simulink model "ButtonLogic"  (R2023b)
settings: Solver=FixedStepDiscrete  StartTime=0.0  StopTime=inf  FixedStep=0.005  RelTol=1e-3  EnableMultiTasking=on
model workspace (MAT data in the model file):
  inSetButton = 0
undefined symbols (not defined in the file or in its folder): eStateName
libraries: simulink x5
(part 1 of 3)
settings Model: DataDictionary=ButtonLogicData.sldd  Creator=pkpam  LastModifiedBy=pkpam
settings SolverCC: AlgebraicLoopSolver=TrustRegion  AutoInsertRateTranBlk=on
settings DataIOCC: LimitDataPoints=on
settings OptimizationCC: DefaultUnderspecifiedDataType=single  ReuseModelBlockBuffer=off  PassReuseOutputArgsAs=Individual arguments  ZeroExternalMemoryAtStartup=off  ZeroInternalMemoryAtStartup=off  OptimizationLevel=level1  EfficientTunableParamExpr=on
settings DebuggingCC: ParameterTunabilityLossMsg=error  UnconnectedInputMsg=warning  UnconnectedOutputMsg=warning  UnconnectedLineMsg=warning  AssertControl=DisableAll  AllowSymbolicDim=off  SFUnexpectedBacktrackingDiag=warning  SFNoUnconditionalDefaultTransitionDiag=warning  SFExecutionAtInitializationDiag=none  ArithmeticOperatorsInVariantConditions=warning
settings ModelReferenceCC: EnableRefExpFcnMdlSchedulingChecks=on  ModelReferenceNumInstancesAllowed=Single
settings SFSimCC: SimUseLocalCustomCode=off  MATLABDynamicMemAlloc=off  CustomCodeUndefinedFunction=UseInterfaceOnly
settings RTWCC: Description=Embedded Coder  SystemTargetFile=ert.tlc  TemplateMakefile=ert_default_tmf  GenerateReport=on  RTWUseLocalCustomCode=off  Toolchain=LCC-win64 v2.4.1 | gmake (64-bit Windows)  DataTypeReplacement=CDataTypesFixedWidth  GenerateWebview=on  CheckMdlBeforeBuild=Warning  DLArmComputeVersion=19.05
settings CodeAppCC: ForceParamTrailComments=on  IgnoreCustomStorageClasses=off  OperatorAnnotations=on  SimulinkDataObjDesc=on  SFDataObjDesc=on  MATLABFcnDesc=on  InsertBlockDesc=on  StateflowObjectComments=on
settings ERTTargetCC: UtilityFuncGeneration=Shared location  GenerateSampleERTMain=on  SupportNonFinite=off  GenerateSharedConstants=off  MultiInstanceErrorCode=Warning  ERTCustomFileTemplate=example_file_process.tlc  GlobalDataDefinition=InSourceFile  ERTFilePackagingFormat=CompactWithDataFile  IndentSize=4  MaxIdInt64=INT64_MAX  MinIdInt64=INT64_MIN  MaxIdUint64=UINT64_MAX  MaxIdInt32=INT32_MAX  MinIdInt32=INT32_MIN  MaxIdUint32=UINT32_MAX  MaxIdInt16=INT16_MAX  MinIdInt16=INT16_MIN  MaxIdUint16=UINT16_MAX  MaxIdInt8=INT8_MAX  MinIdInt8=INT8_MIN  MaxIdUint8=UINT8_MAX
settings ConfigComp: CovMetricSettings=dw  CovSaveCumulativeToWorkspaceVar=on  CovSaveSingleToWorkspaceVar=on  CovExternalEMLEnable=off  CovSFcnEnable=off

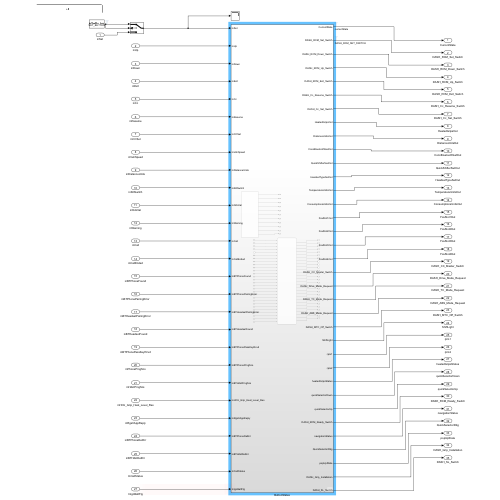
[thumbnail: Simulink's stored preview of the top-level diagram]
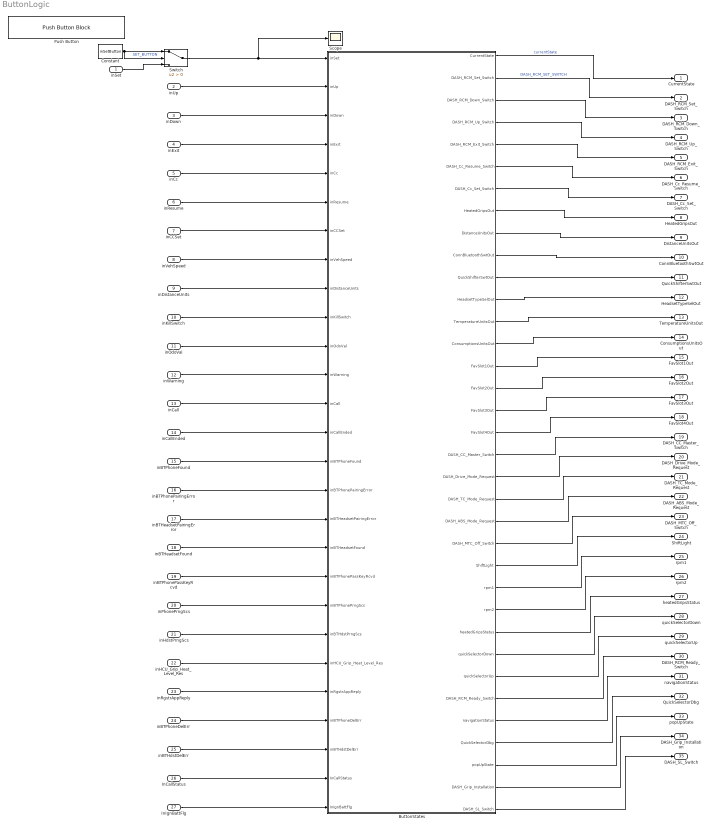
== system ButtonLogic ==
  inSet : Inport  OutDataTypeStr=boolean
  inUp : Inport  Port=2  OutDataTypeStr=boolean
  inDown : Inport  Port=3  OutDataTypeStr=boolean
  inExit : Inport  Port=4  OutDataTypeStr=boolean
  inCc : Inport  Port=5
  inResume : Inport  Port=6
  inCCSet : Inport  Port=7
  inVehSpeed : Inport  Port=8
  inDistanceUnits : Inport  Port=9  OutDataTypeStr=uint8
  inKillSwitch : Inport  Port=10  OutDataTypeStr=uint8
  inOdoVal : Inport  Port=11  OutDataTypeStr=uint32
  inWarning : Inport  Port=12
  inCall : Inport  Port=13
  inCallEnded : Inport  Port=14
  inBTPhoneFound : Inport  Port=15  OutDataTypeStr=boolean
  inBTPhonePairingError : Inport  Port=16  OutDataTypeStr=boolean
  inBTHeadsetPairingError : Inport  Port=17  OutDataTypeStr=boolean
  inBTHeadsetFound : Inport  Port=18  OutDataTypeStr=boolean
  inBTPhonePassKeyRcvd : Inport  Port=19  OutDataTypeStr=boolean
  inPhonePrngScs : Inport  Port=20  OutDataTypeStr=boolean
  inHdstPrngScs : Inport  Port=21  OutDataTypeStr=boolean
  inHCU_Grip_Heat_Level_Res : Inport  Port=22  OutDataTypeStr=boolean
  inRgstrAppReply : Inport  Port=23  OutDataTypeStr=boolean
  inBTPhoneDelErr : Inport  Port=24  OutDataTypeStr=boolean
  inBTHdstDelErr : Inport  Port=25  OutDataTypeStr=boolean
  InCallStatus : Inport  Port=26  OutDataTypeStr=uint8
  InIgnBattFlg : Inport  Port=27  OutDataTypeStr=boolean
  ButtonStates : Subsystem
  Constant : Constant  Value=inSetButton  OutDataTypeStr=boolean
  Push Button : PushButtonBlock  ButtonText=SET  OffValue=0.000000
  Scope : Scope
  Switch : Switch  Criteria=u2 > Threshold  SaturateOnIntegerOverflow=off  InputSameDT=off
  CurrentState : Outport
  DASH_RCM_Set_Switch : Outport  Port=2
  DASH_RCM_Down_Switch : Outport  Port=3
  DASH_RCM_Up_Switch : Outport  Port=4
  DASH_RCM_Exit_Switch : Outport  Port=5
  DASH_Cc_Resume_Switch : Outport  Port=6
  DASH_Cc_Set_Switch : Outport  Port=7
  HeatedGripsOut : Outport  Port=8
  DistanceUnitsOut : Outport  Port=9
  ConnBluetoothSwtOut : Outport  Port=10
  QuickShifterSwtOut : Outport  Port=11
  HeadsetTypeSelOut : Outport  Port=12
  TemperatureUnitsOut : Outport  Port=13
  ConsumptionsUnitsOut : Outport  Port=14
  FavSlot1Out : Outport  Port=15
  FavSlot2Out : Outport  Port=16
  FavSlot3Out : Outport  Port=17
  FavSlot4Out : Outport  Port=18
  DASH_CC_Master_Switch : Outport  Port=19
  DASH_Drive_Mode_Request : Outport  Port=20
  DASH_TC_Mode_Request : Outport  Port=21
  DASH_ABS_Mode_Request : Outport  Port=22
  DASH_MTC_Off_Switch : Outport  Port=23
  ShiftLight : Outport  Port=24
  rpm1 : Outport  Port=25
  rpm2 : Outport  Port=26
  heatedGripsStatus : Outport  Port=27
  quickSelectorDown : Outport  Port=28
  quickSelectorUp : Outport  Port=29
  DASH_RCM_Ready_Switch : Outport  Port=30
  navigationStatus : Outport  Port=31
  QuickSelectorDbg : Outport  Port=32
  popUpState : Outport  Port=33
  DASH_Grip_Installation : Outport  Port=34
  DASH_SL_Switch : Outport  Port=35  OutDataTypeStr=uint8
  wires:
  ButtonStates/16(FavSlot2Out) -> FavSlot2Out/1
  Constant/1 -> Switch/2, Switch/1  "SET_BUTTON"
  inCc/1 -> ButtonStates/5(inCc)
  ButtonStates/11(QuickShifterSwtOut) -> QuickShifterSwtOut/1
  inBTPhoneDelErr/1 -> ButtonStates/24(inBTPhoneDelErr)
  inVehSpeed/1 -> ButtonStates/8(inVehSpeed)
  inDown/1 -> ButtonStates/3(inDown)
  Switch/1 -> Scope/1, ButtonStates/1(inSet)
  ButtonStates/21(DASH_TC_Mode_Request) -> DASH_TC_Mode_Request/1
  ButtonStates/10(ConnBluetoothSwtOut) -> ConnBluetoothSwtOut/1
  inBTPhonePairingError/1 -> ButtonStates/16(inBTPhonePairingError)
  inExit/1 -> ButtonStates/4(inExit)
  ButtonStates/32(QuickSelectorDbg) -> QuickSelectorDbg/1
  inHdstPrngScs/1 -> ButtonStates/21(inBTHdstPrngScs)
  inCall/1 -> ButtonStates/13(inCall)
  inSet/1 -> Switch/3
  ButtonStates/34(DASH_Grip_Installation) -> DASH_Grip_Installation/1
  ButtonStates/13(TemperatureUnitsOut) -> TemperatureUnitsOut/1
  ButtonStates/9(DistanceUnitsOut) -> DistanceUnitsOut/1
  inUp/1 -> ButtonStates/2(inUp)
  ButtonStates/19(DASH_CC_Master_Switch) -> DASH_CC_Master_Switch/1
  ButtonStates/12(HeadsetTypeSelOut) -> HeadsetTypeSelOut/1
  inHCU_Grip_Heat_Level_Res/1 -> ButtonStates/22(inHCU_Grip_Heat_Level_Res)
  inResume/1 -> ButtonStates/6(inResume)
  ButtonStates/24(ShiftLight) -> ShiftLight/1
  ButtonStates/18(FavSlot4Out) -> FavSlot4Out/1
  ButtonStates/1(CurrentState) -> CurrentState/1  "currentState"
  inCCSet/1 -> ButtonStates/7(inCCSet)
  ButtonStates/7(DASH_Cc_Set_Switch) -> DASH_Cc_Set_Switch/1
  ButtonStates/3(DASH_RCM_Down_Switch) -> DASH_RCM_Down_Switch/1
  inCallEnded/1 -> ButtonStates/14(inCallEnded)
  inDistanceUnits/1 -> ButtonStates/9(inDistanceUnits)
  ButtonStates/5(DASH_RCM_Exit_Switch) -> DASH_RCM_Exit_Switch/1
  inKillSwitch/1 -> ButtonStates/10(inKillSwitch)
  ButtonStates/20(DASH_Drive_Mode_Request) -> DASH_Drive_Mode_Request/1
  inBTHeadsetFound/1 -> ButtonStates/18(inBTHeadsetFound)
  inBTHeadsetPairingError/1 -> ButtonStates/17(inBTHeadsetPairingError)
  inOdoVal/1 -> ButtonStates/11(inOdoVal)
  ButtonStates/31(navigationStatus) -> navigationStatus/1
  ButtonStates/25(rpm1) -> rpm1/1
  ButtonStates/22(DASH_ABS_Mode_Request) -> DASH_ABS_Mode_Request/1
  inWarning/1 -> ButtonStates/12(inWarning)
  ButtonStates/33(popUpState) -> popUpState/1
  ButtonStates/28(quickSelectorDown) -> quickSelectorDown/1
  ButtonStates/6(DASH_Cc_Resume_Switch) -> DASH_Cc_Resume_Switch/1
  inBTPhoneFound/1 -> ButtonStates/15(inBTPhoneFound)
  ButtonStates/4(DASH_RCM_Up_Switch) -> DASH_RCM_Up_Switch/1
  ButtonStates/2(DASH_RCM_Set_Switch) -> DASH_RCM_Set_Switch/1  "DASH_RCM_SET_SWITCH"
  inBTHdstDelErr/1 -> ButtonStates/25(inBTHdstDelErr)
  inBTPhonePassKeyRcvd/1 -> ButtonStates/19(inBTPhonePassKeyRcvd)
  inRgstrAppReply/1 -> ButtonStates/23(inRgstrAppReply)
  inPhonePrngScs/1 -> ButtonStates/20(inBTPhonePrngScs)
  InCallStatus/1 -> ButtonStates/26(InCallStatus)
  ButtonStates/27(heatedGripsStatus) -> heatedGripsStatus/1
  ButtonStates/26(rpm2) -> rpm2/1
  ButtonStates/17(FavSlot3Out) -> FavSlot3Out/1
  ButtonStates/8(HeatedGripsOut) -> HeatedGripsOut/1
  ButtonStates/30(DASH_RCM_Ready_Switch) -> DASH_RCM_Ready_Switch/1
  ButtonStates/23(DASH_MTC_Off_Switch) -> DASH_MTC_Off_Switch/1
  ButtonStates/15(FavSlot1Out) -> FavSlot1Out/1
  ButtonStates/14(ConsumptionsUnitsOut) -> ConsumptionsUnitsOut/1
  ButtonStates/29(quickSelectorUp) -> quickSelectorUp/1
  ButtonStates/35(DASH_SL_Switch) -> DASH_SL_Switch/1
  InIgnBattFlg/1 -> ButtonStates/27(InIgnBattFlg)

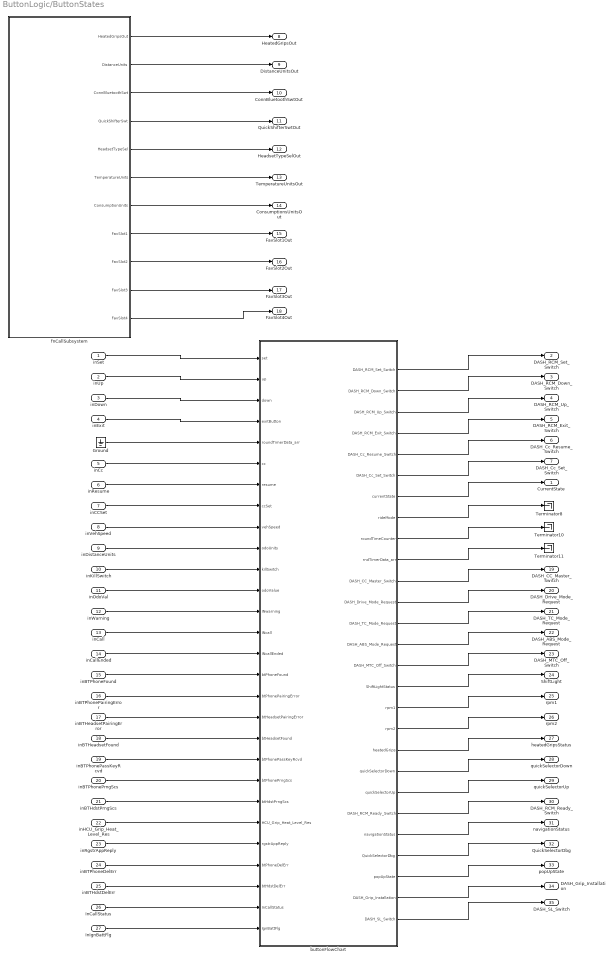
== system ButtonLogic/ButtonStates ==
  inSet : Inport  OutDataTypeStr=boolean
  inUp : Inport  Port=2  OutDataTypeStr=boolean
  inDown : Inport  Port=3  OutDataTypeStr=boolean
  inExit : Inport  Port=4  OutDataTypeStr=boolean
  inCc : Inport  Port=5
  inResume : Inport  Port=6
  inCCSet : Inport  Port=7
  inVehSpeed : Inport  Port=8  OutDataTypeStr=double
  inDistanceUnits : Inport  Port=9
  inKillSwitch : Inport  Port=10
  inOdoVal : Inport  Port=11
  inWarning : Inport  Port=12
  inCall : Inport  Port=13
  inCallEnded : Inport  Port=14  OutDataTypeStr=boolean
  inBTPhoneFound : Inport  Port=15  OutDataTypeStr=boolean
  inBTPhonePairingError : Inport  Port=16  OutDataTypeStr=boolean
  inBTHeadsetPairingError : Inport  Port=17  OutDataTypeStr=boolean
  inBTHeadsetFound : Inport  Port=18  OutDataTypeStr=boolean
  inBTPhonePassKeyRcvd : Inport  Port=19  OutDataTypeStr=boolean
  inBTPhonePrngScs : Inport  Port=20  OutDataTypeStr=boolean
  inBTHdstPrngScs : Inport  Port=21  OutDataTypeStr=boolean
  inHCU_Grip_Heat_Level_Res : Inport  Port=22  OutDataTypeStr=boolean
  inRgstrAppReply : Inport  Port=23  OutDataTypeStr=boolean
  inBTPhoneDelErr : Inport  Port=24  OutDataTypeStr=boolean
  inBTHdstDelErr : Inport  Port=25  OutDataTypeStr=boolean
  InCallStatus : Inport  Port=26  OutDataTypeStr=uint8
  InIgnBattFlg : Inport  Port=27
  Ground : Ground
  Terminator10 : Terminator
  Terminator11 : Terminator
  Terminator8 : Terminator
  buttonFlowChart : Stateflow chart  TreatAsAtomicUnit=on
  fnCallSubsystem : Subsystem
  CurrentState : Outport
  DASH_RCM_Set_Switch : Outport  Port=2
  DASH_RCM_Down_Switch : Outport  Port=3
  DASH_RCM_Up_Switch : Outport  Port=4
  DASH_RCM_Exit_Switch : Outport  Port=5
  DASH_Cc_Resume_Switch : Outport  Port=6
  DASH_Cc_Set_Switch : Outport  Port=7
  HeatedGripsOut : Outport  Port=8
  DistanceUnitsOut : Outport  Port=9
  ConnBluetoothSwtOut : Outport  Port=10
  QuickShifterSwtOut : Outport  Port=11
  HeadsetTypeSelOut : Outport  Port=12
  TemperatureUnitsOut : Outport  Port=13
  ConsumptionsUnitsOut : Outport  Port=14
  FavSlot1Out : Outport  Port=15
  FavSlot2Out : Outport  Port=16
  FavSlot3Out : Outport  Port=17
  FavSlot4Out : Outport  Port=18
  DASH_CC_Master_Switch : Outport  Port=19
  DASH_Drive_Mode_Request : Outport  Port=20
  DASH_TC_Mode_Request : Outport  Port=21
  DASH_ABS_Mode_Request : Outport  Port=22
  DASH_MTC_Off_Switch : Outport  Port=23
  ShiftLight : Outport  Port=24
  rpm1 : Outport  Port=25
  rpm2 : Outport  Port=26
  heatedGripsStatus : Outport  Port=27
  quickSelectorDown : Outport  Port=28
  quickSelectorUp : Outport  Port=29
  DASH_RCM_Ready_Switch : Outport  Port=30
  navigationStatus : Outport  Port=31
  QuickSelectorDbg : Outport  Port=32
  popUpState : Outport  Port=33
  DASH_Grip_Installation : Outport  Port=34
  DASH_SL_Switch : Outport  Port=35  OutDataTypeStr=uint8
  wires:
  buttonFlowChart/14(DASH_ABS_Mode_Request) -> DASH_ABS_Mode_Request/1
  fnCallSubsystem/9(FavSlot2) -> FavSlot2Out/1
  fnCallSubsystem/3(ConnBluetoothSwt) -> ConnBluetoothSwtOut/1
  fnCallSubsystem/1(HeatedGripsOut) -> HeatedGripsOut/1
  fnCallSubsystem/2(DistanceUnits) -> DistanceUnitsOut/1
  fnCallSubsystem/7(ConsumptionUnits) -> ConsumptionsUnitsOut/1
  fnCallSubsystem/5(HeadsetTypeSel) -> HeadsetTypeSelOut/1
  fnCallSubsystem/4(QuickShifterSwt) -> QuickShifterSwtOut/1
  fnCallSubsystem/6(TemperatureUnits) -> TemperatureUnitsOut/1
  buttonFlowChart/4(DASH_RCM_Exit_Switch) -> DASH_RCM_Exit_Switch/1
  inExit/1 -> buttonFlowChart/4(exitButton)
  fnCallSubsystem/8(FavSlot1) -> FavSlot1Out/1
  fnCallSubsystem/10(FavSlot3) -> FavSlot3Out/1
  fnCallSubsystem/11(FavSlot4) -> FavSlot4Out/1
  inCCSet/1 -> buttonFlowChart/8(ccSet)
  inSet/1 -> buttonFlowChart/1(set)
  inUp/1 -> buttonFlowChart/2(up)
  inDown/1 -> buttonFlowChart/3(down)
  buttonFlowChart/10(rndTimerData_arr) -> Terminator11/1
  Ground/1 -> buttonFlowChart/5(roundTimerData_arr)
  inCc/1 -> buttonFlowChart/6(cc)
  buttonFlowChart/25(popUpState) -> popUpState/1
  inResume/1 -> buttonFlowChart/7(resume)
  inVehSpeed/1 -> buttonFlowChart/9(vehSpeed)
  inDistanceUnits/1 -> buttonFlowChart/10(odoUnits)
  inBTHdstPrngScs/1 -> buttonFlowChart/22(btHdstPrngScs)
  inKillSwitch/1 -> buttonFlowChart/11(killSwitch)
  buttonFlowChart/1(DASH_RCM_Set_Switch) -> DASH_RCM_Set_Switch/1
  inHCU_Grip_Heat_Level_Res/1 -> buttonFlowChart/23(HCU_Grip_Heat_Level_Res)
  inOdoVal/1 -> buttonFlowChart/12(odoValue)
  buttonFlowChart/5(DASH_Cc_Resume_Switch) -> DASH_Cc_Resume_Switch/1
  inWarning/1 -> buttonFlowChart/13(INwarning)
  inCall/1 -> buttonFlowChart/14(INcall)
  buttonFlowChart/13(DASH_TC_Mode_Request) -> DASH_TC_Mode_Request/1
  buttonFlowChart/3(DASH_RCM_Up_Switch) -> DASH_RCM_Up_Switch/1
  inCallEnded/1 -> buttonFlowChart/15(INcallEnded)
  buttonFlowChart/20(quickSelectorDown) -> quickSelectorDown/1
  buttonFlowChart/16(ShiftLightStatus) -> ShiftLight/1
  inBTPhoneFound/1 -> buttonFlowChart/16(btPhoneFound)
  inBTPhonePairingError/1 -> buttonFlowChart/17(btPhonePairingError)
  buttonFlowChart/26(DASH_Grip_Installation) -> DASH_Grip_Installation/1
  buttonFlowChart/17(rpm1) -> rpm1/1
  buttonFlowChart/2(DASH_RCM_Down_Switch) -> DASH_RCM_Down_Switch/1
  inBTHeadsetPairingError/1 -> buttonFlowChart/18(btHeadsetPairingError)
  buttonFlowChart/18(rpm2) -> rpm2/1
  inBTHeadsetFound/1 -> buttonFlowChart/19(btHeadsetFound)
  inBTPhonePassKeyRcvd/1 -> buttonFlowChart/20(btPhonePassKeyRcvd)
  inBTPhonePrngScs/1 -> buttonFlowChart/21(btPhonePrngScs)
  buttonFlowChart/11(DASH_CC_Master_Switch) -> DASH_CC_Master_Switch/1
  inRgstrAppReply/1 -> buttonFlowChart/24(rgstrAppReply)
  buttonFlowChart/19(heatedGrips) -> heatedGripsStatus/1
  inBTPhoneDelErr/1 -> buttonFlowChart/25(btPhoneDelErr)
  inBTHdstDelErr/1 -> buttonFlowChart/26(btHdstDelErr)
  buttonFlowChart/6(DASH_Cc_Set_Switch) -> DASH_Cc_Set_Switch/1
  buttonFlowChart/7(currentState) -> CurrentState/1
  buttonFlowChart/8(rideMode) -> Terminator8/1
  buttonFlowChart/9(roundTimeCounter) -> Terminator10/1
  buttonFlowChart/21(quickSelectorUp) -> quickSelectorUp/1
  buttonFlowChart/12(DASH_Drive_Mode_Request) -> DASH_Drive_Mode_Request/1
  buttonFlowChart/15(DASH_MTC_Off_Switch) -> DASH_MTC_Off_Switch/1
  buttonFlowChart/22(DASH_RCM_Ready_Switch) -> DASH_RCM_Ready_Switch/1
  buttonFlowChart/23(navigationStatus) -> navigationStatus/1
  buttonFlowChart/24(QuickSelectorDbg) -> QuickSelectorDbg/1
  InCallStatus/1 -> buttonFlowChart/27(InCallStatus)
  buttonFlowChart/27(DASH_SL_Switch) -> DASH_SL_Switch/1
  InIgnBattFlg/1 -> buttonFlowChart/28(IgnBattFlg)

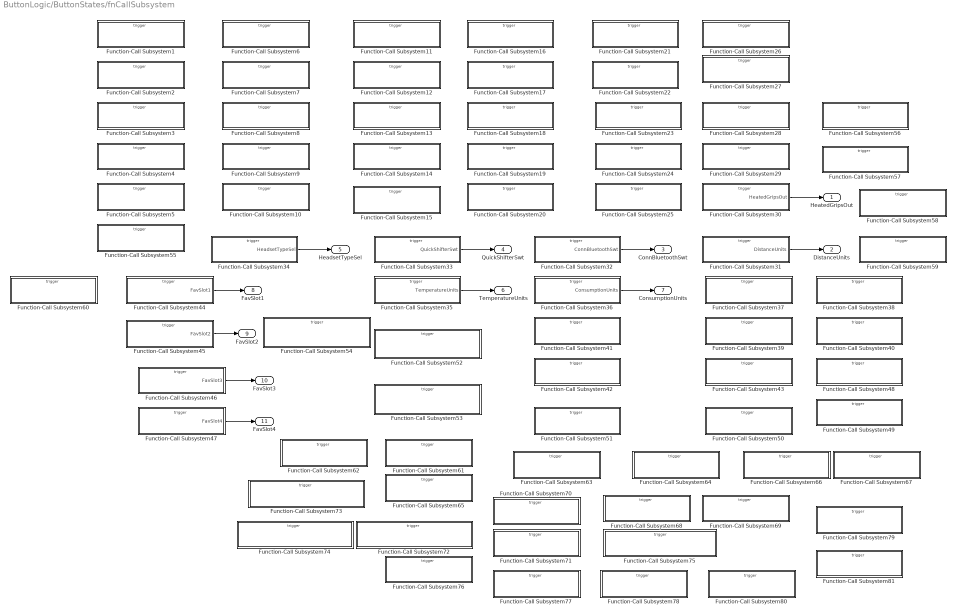
== system ButtonLogic/ButtonStates/fnCallSubsystem ==
  Function-Call Subsystem1 : Subsystem  TreatAsAtomicUnit=on
  Function-Call Subsystem10 : Subsystem  TreatAsAtomicUnit=on
  Function-Call Subsystem11 : Subsystem  TreatAsAtomicUnit=on
  Function-Call Subsystem12 : Subsystem  TreatAsAtomicUnit=on
  Function-Call Subsystem13 : Subsystem  TreatAsAtomicUnit=on
  Function-Call Subsystem14 : Subsystem  TreatAsAtomicUnit=on
  Function-Call Subsystem15 : Subsystem  TreatAsAtomicUnit=on
  Function-Call Subsystem16 : Subsystem  TreatAsAtomicUnit=on
  Function-Call Subsystem17 : Subsystem  TreatAsAtomicUnit=on
  Function-Call Subsystem18 : Subsystem  TreatAsAtomicUnit=on
  Function-Call Subsystem19 : Subsystem  TreatAsAtomicUnit=on
  Function-Call Subsystem2 : Subsystem  TreatAsAtomicUnit=on
  Function-Call Subsystem20 : Subsystem  TreatAsAtomicUnit=on
  Function-Call Subsystem21 : Subsystem  TreatAsAtomicUnit=on
  Function-Call Subsystem22 : Subsystem  TreatAsAtomicUnit=on
  Function-Call Subsystem23 : Subsystem  TreatAsAtomicUnit=on
  Function-Call Subsystem24 : Subsystem  TreatAsAtomicUnit=on
  Function-Call Subsystem25 : Subsystem  TreatAsAtomicUnit=on
  Function-Call Subsystem26 : Subsystem  TreatAsAtomicUnit=on
  Function-Call Subsystem27 : Subsystem  TreatAsAtomicUnit=on
  Function-Call Subsystem28 : Subsystem  TreatAsAtomicUnit=on
  Function-Call Subsystem29 : Subsystem  TreatAsAtomicUnit=on
  Function-Call Subsystem3 : Subsystem  TreatAsAtomicUnit=on
  Function-Call Subsystem30 : Subsystem  TreatAsAtomicUnit=on
  Function-Call Subsystem31 : Subsystem  TreatAsAtomicUnit=on
  Function-Call Subsystem32 : Subsystem  TreatAsAtomicUnit=on
  Function-Call Subsystem33 : Subsystem  TreatAsAtomicUnit=on
  Function-Call Subsystem34 : Subsystem  TreatAsAtomicUnit=on
  Function-Call Subsystem35 : Subsystem  TreatAsAtomicUnit=on
  Function-Call Subsystem36 : Subsystem  TreatAsAtomicUnit=on
  Function-Call Subsystem37 : Subsystem  TreatAsAtomicUnit=on
  Function-Call Subsystem38 : Subsystem  TreatAsAtomicUnit=on
  Function-Call Subsystem39 : Subsystem  TreatAsAtomicUnit=on
  Function-Call Subsystem4 : Subsystem  TreatAsAtomicUnit=on
  Function-Call Subsystem40 : Subsystem  TreatAsAtomicUnit=on
  Function-Call Subsystem41 : Subsystem  TreatAsAtomicUnit=on
  Function-Call Subsystem42 : Subsystem  TreatAsAtomicUnit=on
  Function-Call Subsystem43 : Subsystem  TreatAsAtomicUnit=on
  Function-Call Subsystem44 : Subsystem  TreatAsAtomicUnit=on
  Function-Call Subsystem45 : Subsystem  TreatAsAtomicUnit=on
  Function-Call Subsystem46 : Subsystem  TreatAsAtomicUnit=on
  Function-Call Subsystem47 : Subsystem  TreatAsAtomicUnit=on
  Function-Call Subsystem48 : Subsystem  TreatAsAtomicUnit=on
  Function-Call Subsystem49 : Subsystem  TreatAsAtomicUnit=on
  Function-Call Subsystem5 : Subsystem  TreatAsAtomicUnit=on
  Function-Call Subsystem50 : Subsystem  TreatAsAtomicUnit=on
  Function-Call Subsystem51 : Subsystem  TreatAsAtomicUnit=on
  Function-Call Subsystem52 : Subsystem  TreatAsAtomicUnit=on
  Function-Call Subsystem53 : Subsystem  TreatAsAtomicUnit=on
  Function-Call Subsystem54 : Subsystem  TreatAsAtomicUnit=on
  Function-Call Subsystem55 : Subsystem  TreatAsAtomicUnit=on
  Function-Call Subsystem56 : Subsystem  TreatAsAtomicUnit=on
  Function-Call Subsystem57 : Subsystem  TreatAsAtomicUnit=on
  Function-Call Subsystem58 : Subsystem  TreatAsAtomicUnit=on
  Function-Call Subsystem59 : Subsystem  TreatAsAtomicUnit=on
  Function-Call Subsystem6 : Subsystem  TreatAsAtomicUnit=on
  Function-Call Subsystem60 : Subsystem  TreatAsAtomicUnit=on
  Function-Call Subsystem61 : Subsystem  TreatAsAtomicUnit=on
  Function-Call Subsystem62 : Subsystem  TreatAsAtomicUnit=on
  Function-Call Subsystem63 : Subsystem  TreatAsAtomicUnit=on
  Function-Call Subsystem64 : Subsystem  TreatAsAtomicUnit=on
  Function-Call Subsystem65 : Subsystem  TreatAsAtomicUnit=on
  Function-Call Subsystem66 : Subsystem  TreatAsAtomicUnit=on
  Function-Call Subsystem67 : Subsystem  TreatAsAtomicUnit=on
  Function-Call Subsystem68 : Subsystem  TreatAsAtomicUnit=on
  Function-Call Subsystem69 : Subsystem  TreatAsAtomicUnit=on
  Function-Call Subsystem7 : Subsystem  TreatAsAtomicUnit=on
  Function-Call Subsystem70 : Subsystem  TreatAsAtomicUnit=on
  Function-Call Subsystem71 : Subsystem  TreatAsAtomicUnit=on
  Function-Call Subsystem72 : Subsystem  TreatAsAtomicUnit=on
  Function-Call Subsystem73 : Subsystem  TreatAsAtomicUnit=on
  Function-Call Subsystem74 : Subsystem  TreatAsAtomicUnit=on
  Function-Call Subsystem75 : Subsystem  TreatAsAtomicUnit=on
  Function-Call Subsystem76 : Subsystem  TreatAsAtomicUnit=on
  Function-Call Subsystem77 : Subsystem  TreatAsAtomicUnit=on
  Function-Call Subsystem78 : Subsystem  TreatAsAtomicUnit=on
  Function-Call Subsystem79 : Subsystem  TreatAsAtomicUnit=on
  Function-Call Subsystem8 : Subsystem  TreatAsAtomicUnit=on
  Function-Call Subsystem80 : Subsystem  TreatAsAtomicUnit=on
  Function-Call Subsystem81 : Subsystem  TreatAsAtomicUnit=on
  Function-Call Subsystem9 : Subsystem  TreatAsAtomicUnit=on
  HeatedGripsOut : Outport
  DistanceUnits : Outport  Port=2
  ConnBluetoothSwt : Outport  Port=3
  QuickShifterSwt : Outport  Port=4
  HeadsetTypeSel : Outport  Port=5
  TemperatureUnits : Outport  Port=6
  ConsumptionUnits : Outport  Port=7
  FavSlot1 : Outport  Port=8
  FavSlot2 : Outport  Port=9
  FavSlot3 : Outport  Port=10
  FavSlot4 : Outport  Port=11
  wires:
  Function-Call Subsystem30/1(HeatedGripsOut) -> HeatedGripsOut/1
  Function-Call Subsystem31/1(DistanceUnits) -> DistanceUnits/1
  Function-Call Subsystem32/1(ConnBluetoothSwt) -> ConnBluetoothSwt/1
  Function-Call Subsystem33/1(QuickShifterSwt) -> QuickShifterSwt/1
  Function-Call Subsystem34/1(HeadsetTypeSel) -> HeadsetTypeSel/1
  Function-Call Subsystem35/1(TemperatureUnits) -> TemperatureUnits/1
  Function-Call Subsystem36/1(ConsumptionUnits) -> ConsumptionUnits/1
  Function-Call Subsystem44/1(FavSlot1) -> FavSlot1/1
  Function-Call Subsystem45/1(FavSlot2) -> FavSlot2/1
  Function-Call Subsystem46/1(FavSlot3) -> FavSlot3/1
  Function-Call Subsystem47/1(FavSlot4) -> FavSlot4/1

== system ButtonLogic/ButtonStates/fnCallSubsystem/Function-Call Subsystem1 ==
  BLU_FnRLRndTmrUp : TriggerPort  TriggerType=function-call  IsSimulinkFunction=on  FunctionName=BLU_FnRLRndTmrUp  VariantControl=(inherit)

== system ButtonLogic/ButtonStates/fnCallSubsystem/Function-Call Subsystem10 ==
  BLU_FnCCSwtONCrsCtrl : TriggerPort  TriggerType=function-call  IsSimulinkFunction=on  FunctionName=BLU_FnCCSwtONCrsCtrl  VariantControl=(inherit)

== system ButtonLogic/ButtonStates/fnCallSubsystem/Function-Call Subsystem11 ==
  BLU_FnAudioVolUp : TriggerPort  TriggerType=function-call  IsSimulinkFunction=on  FunctionName=BLU_FnAudioVolUp  VariantControl=(inherit)

== system ButtonLogic/ButtonStates/fnCallSubsystem/Function-Call Subsystem12 ==
  BLU_FnAudioVolDwn : TriggerPort  TriggerType=function-call  IsSimulinkFunction=on  FunctionName=BLU_FnAudioVolDwn  VariantControl=(inherit)

== system ButtonLogic/ButtonStates/fnCallSubsystem/Function-Call Subsystem13 ==
  BLU_FnAudioTglPlayPause : TriggerPort  TriggerType=function-call  IsSimulinkFunction=on  FunctionName=BLU_FnAudioTglPlayPause  VariantControl=(inherit)

== system ButtonLogic/ButtonStates/fnCallSubsystem/Function-Call Subsystem14 ==
  BLU_FnAudioPrevTrack : TriggerPort  TriggerType=function-call  IsSimulinkFunction=on  FunctionName=BLU_FnAudioPrevTrack  VariantControl=(inherit)

== system ButtonLogic/ButtonStates/fnCallSubsystem/Function-Call Subsystem15 ==
  BLU_FnAudioNextTrack : TriggerPort  TriggerType=function-call  IsSimulinkFunction=on  FunctionName=BLU_FnAudioNextTrack  VariantControl=(inherit)

== system ButtonLogic/ButtonStates/fnCallSubsystem/Function-Call Subsystem16 ==
  BLU_FnNavVolUp : TriggerPort  TriggerType=function-call  IsSimulinkFunction=on  FunctionName=BLU_FnNavVolUp  VariantControl=(inherit)

== system ButtonLogic/ButtonStates/fnCallSubsystem/Function-Call Subsystem17 ==
  BLU_FnNavVolDwn : TriggerPort  TriggerType=function-call  IsSimulinkFunction=on  FunctionName=BLU_FnNavVolDwn  VariantControl=(inherit)

== system ButtonLogic/ButtonStates/fnCallSubsystem/Function-Call Subsystem18 ==
  BLU_FnClkSaveTime : TriggerPort  TriggerType=function-call  IsSimulinkFunction=on  FunctionName=BLU_FnClkSaveTime  VariantControl=(inherit)

== system ButtonLogic/ButtonStates/fnCallSubsystem/Function-Call Subsystem19 ==
  BLU_FnClkIncHrs : TriggerPort  TriggerType=function-call  IsSimulinkFunction=on  FunctionName=BLU_FnClkIncHrs  VariantControl=(inherit)
  Terminator : Terminator
  u : ArgIn  ArgumentName=u
  wires:
  u/1 -> Terminator/1

== system ButtonLogic/ButtonStates/fnCallSubsystem/Function-Call Subsystem2 ==
  BLU_FnRLRndTmrDwn : TriggerPort  TriggerType=function-call  IsSimulinkFunction=on  FunctionName=BLU_FnRLRndTmrDwn  VariantControl=(inherit)

== system ButtonLogic/ButtonStates/fnCallSubsystem/Function-Call Subsystem20 ==
  BLU_FnClkDecHrs : TriggerPort  TriggerType=function-call  IsSimulinkFunction=on  FunctionName=BLU_FnClkDecHrs  VariantControl=(inherit)
  Terminator : Terminator
  u : ArgIn  ArgumentName=u
  wires:
  u/1 -> Terminator/1

== system ButtonLogic/ButtonStates/fnCallSubsystem/Function-Call Subsystem21 ==
  BLU_FnClkIncMins : TriggerPort  TriggerType=function-call  IsSimulinkFunction=on  FunctionName=BLU_FnClkIncMins  VariantControl=(inherit)
  Terminator : Terminator
  u : ArgIn  ArgumentName=u
  wires:
  u/1 -> Terminator/1

== system ButtonLogic/ButtonStates/fnCallSubsystem/Function-Call Subsystem22 ==
  BLU_FnClkDecMins : TriggerPort  TriggerType=function-call  IsSimulinkFunction=on  FunctionName=BLU_FnClkDecMins  VariantControl=(inherit)
  Terminator : Terminator
  u : ArgIn  ArgumentName=u
  wires:
  u/1 -> Terminator/1

== system ButtonLogic/ButtonStates/fnCallSubsystem/Function-Call Subsystem23 ==
  BLU_FnClkSaveDate : TriggerPort  TriggerType=function-call  IsSimulinkFunction=on  FunctionName=BLU_FnClkSaveDate  VariantControl=(inherit)

== system ButtonLogic/ButtonStates/fnCallSubsystem/Function-Call Subsystem24 ==
  BLU_FnClkIncDateDig3 : TriggerPort  TriggerType=function-call  IsSimulinkFunction=on  FunctionName=BLU_FnClkIncDateDig3  VariantControl=(inherit)

== system ButtonLogic/ButtonStates/fnCallSubsystem/Function-Call Subsystem25 ==
  BLU_FnClkIncDateDig2 : TriggerPort  TriggerType=function-call  IsSimulinkFunction=on  FunctionName=BLU_FnClkIncDateDig2  VariantControl=(inherit)

== system ButtonLogic/ButtonStates/fnCallSubsystem/Function-Call Subsystem26 ==
  BLU_FnClkIncDateDig1 : TriggerPort  TriggerType=function-call  IsSimulinkFunction=on  FunctionName=BLU_FnClkIncDateDig1  VariantControl=(inherit)

== system ButtonLogic/ButtonStates/fnCallSubsystem/Function-Call Subsystem27 ==
  BLU_FnClkDecDateDig3 : TriggerPort  TriggerType=function-call  IsSimulinkFunction=on  FunctionName=BLU_FnClkDecDateDig3  VariantControl=(inherit)

== system ButtonLogic/ButtonStates/fnCallSubsystem/Function-Call Subsystem28 ==
  BLU_FnClkDecDateDig2 : TriggerPort  TriggerType=function-call  IsSimulinkFunction=on  FunctionName=BLU_FnClkDecDateDig2  VariantControl=(inherit)

== system ButtonLogic/ButtonStates/fnCallSubsystem/Function-Call Subsystem29 ==
  BLU_FnClkDecDateDig1 : TriggerPort  TriggerType=function-call  IsSimulinkFunction=on  FunctionName=BLU_FnClkDecDateDig1  VariantControl=(inherit)

== system ButtonLogic/ButtonStates/fnCallSubsystem/Function-Call Subsystem3 ==
  BLU_FnRLResetRndTmr : TriggerPort  TriggerType=function-call  IsSimulinkFunction=on  FunctionName=BLU_FnRLResetRndTmr  VariantControl=(inherit)

== system ButtonLogic/ButtonStates/fnCallSubsystem/Function-Call Subsystem30 ==
  BLU_FnSetHeatedGrips : TriggerPort  TriggerType=function-call  IsSimulinkFunction=on  FunctionName=BLU_FnSetHeatedGrips  VariantControl=(inherit)
  u : ArgIn  OutDataTypeStr=Enum: eStateName  ArgumentName=u
  HeatedGripsOut : Outport
  wires:
  u/1 -> HeatedGripsOut/1

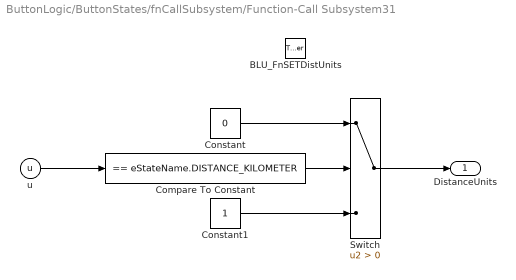
== system ButtonLogic/ButtonStates/fnCallSubsystem/Function-Call Subsystem31 ==
  BLU_FnSETDistUnits : TriggerPort  TriggerType=function-call  IsSimulinkFunction=on  FunctionName=BLU_FnSETDistUnits  VariantControl=(inherit)
  Compare To Constant : simulink/Logic and Bit Operations/Compare To Constant  relop===  const=eStateName.DISTANCE_KILOMETER  OutDataTypeStr=boolean
  Constant : Constant  Value=0  OutDataTypeStr=uint8
  Constant1 : Constant  OutDataTypeStr=uint8
  Switch : Switch  Criteria=u2 > Threshold  SaturateOnIntegerOverflow=off  InputSameDT=off
  u : ArgIn  OutDataTypeStr=Enum: eStateName  ArgumentName=u
  DistanceUnits : Outport
  wires:
  Constant1/1 -> Switch/3
  Constant/1 -> Switch/1
  Compare To Constant/1 -> Switch/2
  u/1 -> Compare To Constant/1
  Switch/1 -> DistanceUnits/1

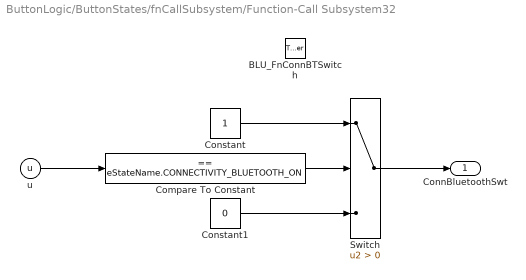
== system ButtonLogic/ButtonStates/fnCallSubsystem/Function-Call Subsystem32 ==
  BLU_FnConnBTSwitch : TriggerPort  TriggerType=function-call  IsSimulinkFunction=on  FunctionName=BLU_FnConnBTSwitch  VariantControl=(inherit)
  Compare To Constant : simulink/Logic and Bit Operations/Compare To Constant  relop===  const=eStateName.CONNECTIVITY_BLUETOOTH_ON  OutDataTypeStr=boolean
  Constant : Constant  OutDataTypeStr=uint8
  Constant1 : Constant  Value=0  OutDataTypeStr=uint8
  Switch : Switch  Criteria=u2 > Threshold  SaturateOnIntegerOverflow=off  InputSameDT=off
  u : ArgIn  OutDataTypeStr=Enum: eStateName  ArgumentName=u
  ConnBluetoothSwt : Outport
  wires:
  Switch/1 -> ConnBluetoothSwt/1
  u/1 -> Compare To Constant/1
  Compare To Constant/1 -> Switch/2
  Constant/1 -> Switch/1
  Constant1/1 -> Switch/3

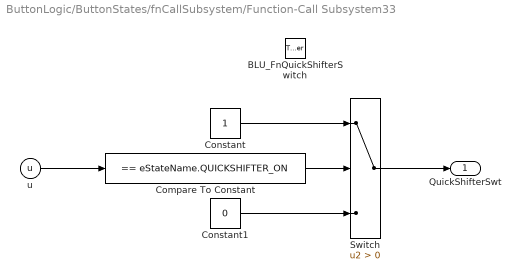
== system ButtonLogic/ButtonStates/fnCallSubsystem/Function-Call Subsystem33 ==
  BLU_FnQuickShifterSwitch : TriggerPort  TriggerType=function-call  IsSimulinkFunction=on  FunctionName=BLU_FnQuickShifterSwitch  VariantControl=(inherit)
  Compare To Constant : simulink/Logic and Bit Operations/Compare To Constant  relop===  const=eStateName.QUICKSHIFTER_ON  OutDataTypeStr=boolean
  Constant : Constant  OutDataTypeStr=uint8
  Constant1 : Constant  Value=0  OutDataTypeStr=uint8
  Switch : Switch  Criteria=u2 > Threshold  SaturateOnIntegerOverflow=off  InputSameDT=off
  u : ArgIn  OutDataTypeStr=Enum: eStateName  ArgumentName=u
  QuickShifterSwt : Outport
  wires:
  Constant1/1 -> Switch/3
  Constant/1 -> Switch/1
  Compare To Constant/1 -> Switch/2
  u/1 -> Compare To Constant/1
  Switch/1 -> QuickShifterSwt/1

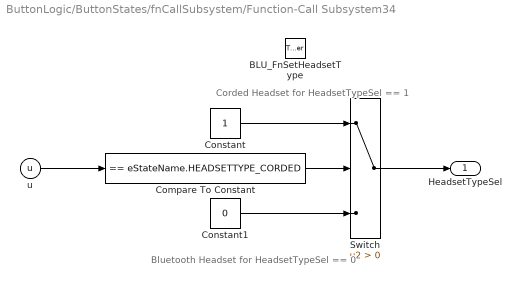
== system ButtonLogic/ButtonStates/fnCallSubsystem/Function-Call Subsystem34 ==
  note: Corded Headset for HeadsetTypeSel == 1
  note: Bluetooth Headset for HeadsetTypeSel == 0
  BLU_FnSetHeadsetType : TriggerPort  TriggerType=function-call  IsSimulinkFunction=on  FunctionName=BLU_FnSetHeadsetType  VariantControl=(inherit)
  Compare To Constant : simulink/Logic and Bit Operations/Compare To Constant  relop===  const=eStateName.HEADSETTYPE_CORDED  OutDataTypeStr=boolean
  Constant : Constant  OutDataTypeStr=uint8
  Constant1 : Constant  Value=0  OutDataTypeStr=uint8
  Switch : Switch  Criteria=u2 > Threshold  SaturateOnIntegerOverflow=off  InputSameDT=off
  u : ArgIn  OutDataTypeStr=Enum: eStateName  ArgumentName=u
  HeadsetTypeSel : Outport
  wires:
  Switch/1 -> HeadsetTypeSel/1
  u/1 -> Compare To Constant/1
  Compare To Constant/1 -> Switch/2
  Constant/1 -> Switch/1
  Constant1/1 -> Switch/3

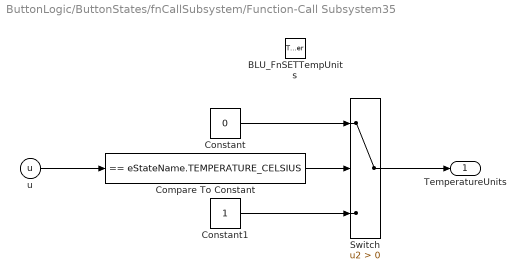
== system ButtonLogic/ButtonStates/fnCallSubsystem/Function-Call Subsystem35 ==
  BLU_FnSETTempUnits : TriggerPort  TriggerType=function-call  IsSimulinkFunction=on  FunctionName=BLU_FnSETTempUnits  VariantControl=(inherit)
  Compare To Constant : simulink/Logic and Bit Operations/Compare To Constant  relop===  const=eStateName.TEMPERATURE_CELSIUS  OutDataTypeStr=boolean
  Constant : Constant  Value=0  OutDataTypeStr=uint8
  Constant1 : Constant  OutDataTypeStr=uint8
  Switch : Switch  Criteria=u2 > Threshold  SaturateOnIntegerOverflow=off  InputSameDT=off
  u : ArgIn  OutDataTypeStr=Enum: eStateName  ArgumentName=u
  TemperatureUnits : Outport
  wires:
  Switch/1 -> TemperatureUnits/1
  u/1 -> Compare To Constant/1
  Compare To Constant/1 -> Switch/2
  Constant/1 -> Switch/1
  Constant1/1 -> Switch/3

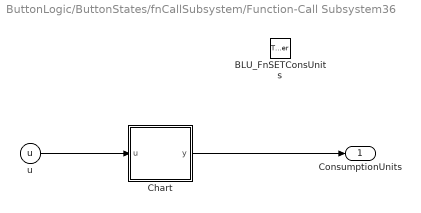
== system ButtonLogic/ButtonStates/fnCallSubsystem/Function-Call Subsystem36 ==
  BLU_FnSETConsUnits : TriggerPort  TriggerType=function-call  IsSimulinkFunction=on  FunctionName=BLU_FnSETConsUnits  VariantControl=(inherit)
  Chart : Stateflow chart  TreatAsAtomicUnit=on
  u : ArgIn  OutDataTypeStr=Enum: eStateName  ArgumentName=u
  ConsumptionUnits : Outport
  wires:
  u/1 -> Chart/1(u)
  Chart/1(y) -> ConsumptionUnits/1

== system ButtonLogic/ButtonStates/fnCallSubsystem/Function-Call Subsystem37 ==
  BLU_FnIncSrvcDistKM : TriggerPort  TriggerType=function-call  IsSimulinkFunction=on  FunctionName=BLU_FnIncSrvcDistKM  VariantControl=(inherit)

== system ButtonLogic/ButtonStates/fnCallSubsystem/Function-Call Subsystem38 ==
  BLU_FnDecSrvcDistKM : TriggerPort  TriggerType=function-call  IsSimulinkFunction=on  FunctionName=BLU_FnDecSrvcDistKM  VariantControl=(inherit)

== system ButtonLogic/ButtonStates/fnCallSubsystem/Function-Call Subsystem39 ==
  BLU_FnIncSrvcDistMI : TriggerPort  TriggerType=function-call  IsSimulinkFunction=on  FunctionName=BLU_FnIncSrvcDistMI  VariantControl=(inherit)

== system ButtonLogic/ButtonStates/fnCallSubsystem/Function-Call Subsystem4 ==
  BLU_FnTIResetTrip1 : TriggerPort  TriggerType=function-call  IsSimulinkFunction=on  FunctionName=BLU_FnTIResetTrip1  VariantControl=(inherit)

== system ButtonLogic/ButtonStates/fnCallSubsystem/Function-Call Subsystem40 ==
  BLU_FnDecSrvcDistMI : TriggerPort  TriggerType=function-call  IsSimulinkFunction=on  FunctionName=BLU_FnDecSrvcDistMI  VariantControl=(inherit)

== system ButtonLogic/ButtonStates/fnCallSubsystem/Function-Call Subsystem41 ==
  BLU_FnDecSrvcMonths : TriggerPort  TriggerType=function-call  IsSimulinkFunction=on  FunctionName=BLU_FnDecSrvcMonths  VariantControl=(inherit)

== system ButtonLogic/ButtonStates/fnCallSubsystem/Function-Call Subsystem42 ==
  BLU_FnIncSrvcMonths : TriggerPort  TriggerType=function-call  IsSimulinkFunction=on  FunctionName=BLU_FnIncSrvcMonths  VariantControl=(inherit)

== system ButtonLogic/ButtonStates/fnCallSubsystem/Function-Call Subsystem43 ==
  BLU_FnSaveSrvcChanges : TriggerPort  TriggerType=function-call  IsSimulinkFunction=on  FunctionName=BLU_FnSaveSrvcChanges  VariantControl=(inherit)

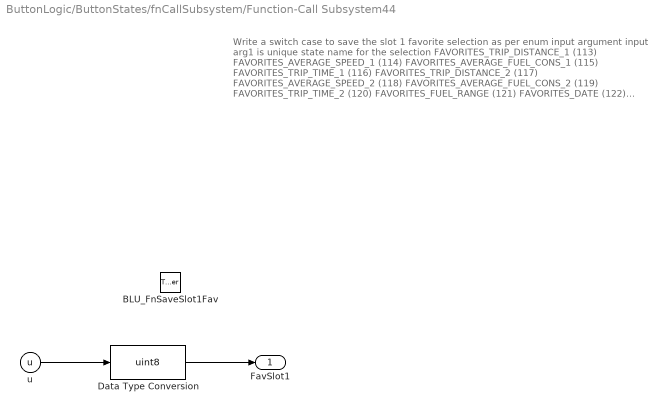
== system ButtonLogic/ButtonStates/fnCallSubsystem/Function-Call Subsystem44 ==
  note: Write a switch case to save the slot 1 favorite selection as per enum input argument
      | input arg1 is unique state name for the selection
      | FAVORITES_TRIP_DISTANCE_1 (113)
      | FAVORITES_AVERAGE_SPEED_1 (114)
      | FAVORITES_AVERAGE_FUEL_CONS_1 (115)
      | FAVORITES_TRIP_TIME_1 (116)
      | FAVORITES_TRIP_DISTANCE_2 (117)
      | FAVORITES_AVERAGE_SPEED_2 (118)
      | FAVORITES_AVERAGE_FUEL_CONS_2 (119)
      | FAVORITES_TRIP_TIME_2 (120)
      | FAVORITES_FUEL_RANGE (121)
      | FAVORITES_DATE (122)
      | FAVORITES_BATTERY (123)
      | FAVORITES_WATER_TEMPERATURE (124)
      | FAVORITES_ODOMETER (125)
      | FAVORITES_SLOT_1 (126)
      | FAVORITES_SLOT_2 (127)
      | FAVORITES_SLOT_3 (128)
      | FAVORITES_SLOT_4 (129)
  BLU_FnSaveSlot1Fav : TriggerPort  TriggerType=function-call  IsSimulinkFunction=on  FunctionName=BLU_FnSaveSlot1Fav  VariantControl=(inherit)
  Data Type Conversion : DataTypeConversion  OutDataTypeStr=uint8  SaturateOnIntegerOverflow=off  RndMeth=Floor
  u : ArgIn  ArgumentName=u
  FavSlot1 : Outport  OutDataTypeStr=uint8
  wires:
  u/1 -> Data Type Conversion/1
  Data Type Conversion/1 -> FavSlot1/1

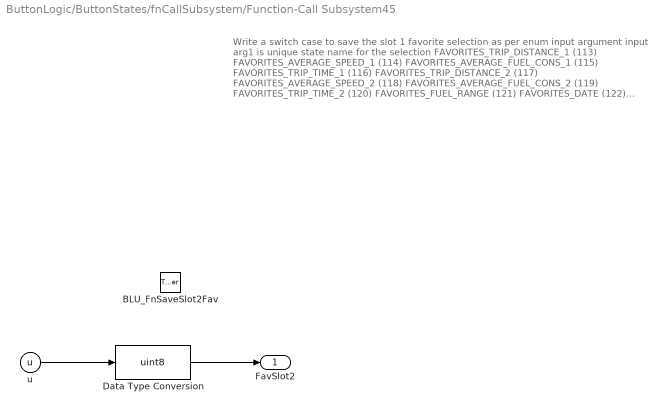
== system ButtonLogic/ButtonStates/fnCallSubsystem/Function-Call Subsystem45 ==
  note: Write a switch case to save the slot 1 favorite selection as per enum input argument
      | input arg1 is unique state name for the selection
      | FAVORITES_TRIP_DISTANCE_1 (113)
      | FAVORITES_AVERAGE_SPEED_1 (114)
      | FAVORITES_AVERAGE_FUEL_CONS_1 (115)
      | FAVORITES_TRIP_TIME_1 (116)
      | FAVORITES_TRIP_DISTANCE_2 (117)
      | FAVORITES_AVERAGE_SPEED_2 (118)
      | FAVORITES_AVERAGE_FUEL_CONS_2 (119)
      | FAVORITES_TRIP_TIME_2 (120)
      | FAVORITES_FUEL_RANGE (121)
      | FAVORITES_DATE (122)
      | FAVORITES_BATTERY (123)
      | FAVORITES_WATER_TEMPERATURE (124)
      | FAVORITES_ODOMETER (125)
      | FAVORITES_SLOT_1 (126)
      | FAVORITES_SLOT_2 (127)
      | FAVORITES_SLOT_3 (128)
      | FAVORITES_SLOT_4 (129)
  BLU_FnSaveSlot2Fav : TriggerPort  TriggerType=function-call  IsSimulinkFunction=on  FunctionName=BLU_FnSaveSlot2Fav  VariantControl=(inherit)
  Data Type Conversion : DataTypeConversion  OutDataTypeStr=uint8  SaturateOnIntegerOverflow=off  RndMeth=Floor
  u : ArgIn  ArgumentName=u
  FavSlot2 : Outport  OutDataTypeStr=uint8
  wires:
  u/1 -> Data Type Conversion/1
  Data Type Conversion/1 -> FavSlot2/1

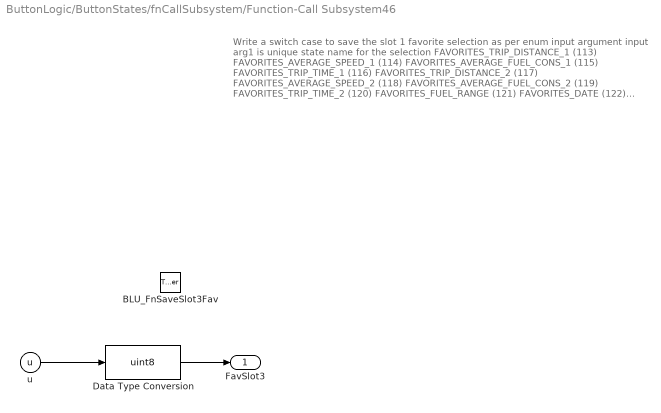
== system ButtonLogic/ButtonStates/fnCallSubsystem/Function-Call Subsystem46 ==
  note: Write a switch case to save the slot 1 favorite selection as per enum input argument
      | input arg1 is unique state name for the selection
      | FAVORITES_TRIP_DISTANCE_1 (113)
      | FAVORITES_AVERAGE_SPEED_1 (114)
      | FAVORITES_AVERAGE_FUEL_CONS_1 (115)
      | FAVORITES_TRIP_TIME_1 (116)
      | FAVORITES_TRIP_DISTANCE_2 (117)
      | FAVORITES_AVERAGE_SPEED_2 (118)
      | FAVORITES_AVERAGE_FUEL_CONS_2 (119)
      | FAVORITES_TRIP_TIME_2 (120)
      | FAVORITES_FUEL_RANGE (121)
      | FAVORITES_DATE (122)
      | FAVORITES_BATTERY (123)
      | FAVORITES_WATER_TEMPERATURE (124)
      | FAVORITES_ODOMETER (125)
      | FAVORITES_SLOT_1 (126)
      | FAVORITES_SLOT_2 (127)
      | FAVORITES_SLOT_3 (128)
      | FAVORITES_SLOT_4 (129)
  BLU_FnSaveSlot3Fav : TriggerPort  TriggerType=function-call  IsSimulinkFunction=on  FunctionName=BLU_FnSaveSlot3Fav  VariantControl=(inherit)
  Data Type Conversion : DataTypeConversion  OutDataTypeStr=uint8  SaturateOnIntegerOverflow=off  RndMeth=Floor
  u : ArgIn  ArgumentName=u
  FavSlot3 : Outport  OutDataTypeStr=uint8
  wires:
  u/1 -> Data Type Conversion/1
  Data Type Conversion/1 -> FavSlot3/1

== system ButtonLogic/ButtonStates/fnCallSubsystem/Function-Call Subsystem47 ==
  note: Write a switch case to save the slot 1 favorite selection as per enum input argument
      | input arg1 is unique state name for the selection
      | FAVORITES_TRIP_DISTANCE_1 (113)
      | FAVORITES_AVERAGE_SPEED_1 (114)
      | FAVORITES_AVERAGE_FUEL_CONS_1 (115)
      | FAVORITES_TRIP_TIME_1 (116)
      | FAVORITES_TRIP_DISTANCE_2 (117)
      | FAVORITES_AVERAGE_SPEED_2 (118)
      | FAVORITES_AVERAGE_FUEL_CONS_2 (119)
      | FAVORITES_TRIP_TIME_2 (120)
      | FAVORITES_FUEL_RANGE (121)
      | FAVORITES_DATE (122)
      | FAVORITES_BATTERY (123)
      | FAVORITES_WATER_TEMPERATURE (124)
      | FAVORITES_ODOMETER (125)
      | FAVORITES_SLOT_1 (126)
      | FAVORITES_SLOT_2 (127)
      | FAVORITES_SLOT_3 (128)
      | FAVORITES_SLOT_4 (129)
  BLU_FnSaveSlot4Fav : TriggerPort  TriggerType=function-call  IsSimulinkFunction=on  FunctionName=BLU_FnSaveSlot4Fav  VariantControl=(inherit)
  Data Type Conversion : DataTypeConversion  OutDataTypeStr=uint8  SaturateOnIntegerOverflow=off  RndMeth=Floor
  u : ArgIn  ArgumentName=u
  FavSlot4 : Outport  OutDataTypeStr=uint8
  wires:
  u/1 -> Data Type Conversion/1
  Data Type Conversion/1 -> FavSlot4/1

== system ButtonLogic/ButtonStates/fnCallSubsystem/Function-Call Subsystem48 ==
  BLU_FnLaunchControlON : TriggerPort  TriggerType=function-call  IsSimulinkFunction=on  FunctionName=BLU_FnLaunchControlON  VariantControl=(inherit)

== system ButtonLogic/ButtonStates/fnCallSubsystem/Function-Call Subsystem49 ==
  BLU_FnLaunchControlOFF : TriggerPort  TriggerType=function-call  IsSimulinkFunction=on  FunctionName=BLU_FnLaunchControlOFF  VariantControl=(inherit)

== system ButtonLogic/ButtonStates/fnCallSubsystem/Function-Call Subsystem5 ==
  BLU_FnTIResetTrip2 : TriggerPort  TriggerType=function-call  IsSimulinkFunction=on  FunctionName=BLU_FnTIResetTrip2  VariantControl=(inherit)

== system ButtonLogic/ButtonStates/fnCallSubsystem/Function-Call Subsystem50 ==
  BLU_FnShiftLightOFF : TriggerPort  TriggerType=function-call  IsSimulinkFunction=on  FunctionName=BLU_FnShiftLightOFF  VariantControl=(inherit)

== system ButtonLogic/ButtonStates/fnCallSubsystem/Function-Call Subsystem51 ==
  BLU_FnShiftLightON : TriggerPort  TriggerType=function-call  IsSimulinkFunction=on  FunctionName=BLU_FnShiftLightON  VariantControl=(inherit)

== system ButtonLogic/ButtonStates/fnCallSubsystem/Function-Call Subsystem52 ==
  BLU_FnSetQuickSelectorUP : TriggerPort  TriggerType=function-call  IsSimulinkFunction=on  FunctionName=BLU_FnSetQuickSelectorUP  VariantControl=(inherit)
  Terminator : Terminator
  u : ArgIn  ArgumentName=u
  wires:
  u/1 -> Terminator/1

== system ButtonLogic/ButtonStates/fnCallSubsystem/Function-Call Subsystem53 ==
  BLU_FnSetQuickSelectorDOWN : TriggerPort  TriggerType=function-call  IsSimulinkFunction=on  FunctionName=BLU_FnSetQuickSelectorDOWN  VariantControl=(inherit)
  Terminator : Terminator
  u : ArgIn  ArgumentName=u
  wires:
  u/1 -> Terminator/1

== system ButtonLogic/ButtonStates/fnCallSubsystem/Function-Call Subsystem54 ==
  BLU_FnNavigationStatus : TriggerPort  TriggerType=function-call  IsSimulinkFunction=on  FunctionName=BLU_FnNavigationStatus  VariantControl=(inherit)
  Terminator : Terminator
  u : ArgIn  ArgumentName=u
  wires:
  u/1 -> Terminator/1

== system ButtonLogic/ButtonStates/fnCallSubsystem/Function-Call Subsystem55 ==
  BLU_FnSETLanguage : TriggerPort  TriggerType=function-call  IsSimulinkFunction=on  FunctionName=BLU_FnSETLanguage  VariantControl=(inherit)
  Terminator : Terminator
  u : ArgIn  OutDataTypeStr=Enum: eStateName  ArgumentName=u
  wires:
  u/1 -> Terminator/1

== system ButtonLogic/ButtonStates/fnCallSubsystem/Function-Call Subsystem56 ==
  BLU_FnTISetAsOvwTrip1 : TriggerPort  TriggerType=function-call  IsSimulinkFunction=on  FunctionName=BLU_FnTISetAsOvwTrip1  VariantControl=(inherit)

== system ButtonLogic/ButtonStates/fnCallSubsystem/Function-Call Subsystem57 ==
  BLU_FnTISetAsOvwTrip2 : TriggerPort  TriggerType=function-call  IsSimulinkFunction=on  FunctionName=BLU_FnTISetAsOvwTrip2  VariantControl=(inherit)

== system ButtonLogic/ButtonStates/fnCallSubsystem/Function-Call Subsystem58 ==
  BLU_FnClkFrmtTgle : TriggerPort  TriggerType=function-call  IsSimulinkFunction=on  FunctionName=BLU_FnClkFrmtTgle  VariantControl=(inherit)
  Terminator : Terminator
  u : ArgIn  OutDataTypeStr=Enum: eStateName  ArgumentName=u
  wires:
  u/1 -> Terminator/1

== system ButtonLogic/ButtonStates/fnCallSubsystem/Function-Call Subsystem59 ==
  BLU_FnDateFrmtTgle : TriggerPort  TriggerType=function-call  IsSimulinkFunction=on  FunctionName=BLU_FnDateFrmtTgle  VariantControl=(inherit)
  Terminator : Terminator
  u : ArgIn  OutDataTypeStr=Enum: eStateName  ArgumentName=u
  wires:
  u/1 -> Terminator/1

== system ButtonLogic/ButtonStates/fnCallSubsystem/Function-Call Subsystem6 ==
  BLU_FnBIWarningsUp : TriggerPort  TriggerType=function-call  IsSimulinkFunction=on  FunctionName=BLU_FnBIWarningsUp  VariantControl=(inherit)

== system ButtonLogic/ButtonStates/fnCallSubsystem/Function-Call Subsystem60 ==
  BLU_FnSetHeatedGripsMode : TriggerPort  TriggerType=function-call  IsSimulinkFunction=on  FunctionName=BLU_FnSetHeatedGripsMode  VariantControl=(inherit)
  Terminator : Terminator
  u : ArgIn  OutDataTypeStr=Enum: eStateName  ArgumentName=u
  wires:
  u/1 -> Terminator/1

== system ButtonLogic/ButtonStates/fnCallSubsystem/Function-Call Subsystem61 ==
  BLU_FnIncomingCallAnswer : TriggerPort  TriggerType=function-call  IsSimulinkFunction=on  FunctionName=BLU_FnIncomingCallAnswer  VariantControl=(inherit)

== system ButtonLogic/ButtonStates/fnCallSubsystem/Function-Call Subsystem62 ==
  BLU_FnIncomingCallReject : TriggerPort  TriggerType=function-call  IsSimulinkFunction=on  FunctionName=BLU_FnIncomingCallReject  VariantControl=(inherit)

== system ButtonLogic/ButtonStates/fnCallSubsystem/Function-Call Subsystem63 ==
  BLU_FnCallVolInc : TriggerPort  TriggerType=function-call  IsSimulinkFunction=on  FunctionName=BLU_FnCallVolInc  VariantControl=(inherit)

== system ButtonLogic/ButtonStates/fnCallSubsystem/Function-Call Subsystem64 ==
  BLU_FnCallVolDec : TriggerPort  TriggerType=function-call  IsSimulinkFunction=on  FunctionName=BLU_FnCallVolDec  VariantControl=(inherit)

== system ButtonLogic/ButtonStates/fnCallSubsystem/Function-Call Subsystem65 ==
  BLU_FnEndCall : TriggerPort  TriggerType=function-call  IsSimulinkFunction=on  FunctionName=BLU_FnEndCall  VariantControl=(inherit)

== system ButtonLogic/ButtonStates/fnCallSubsystem/Function-Call Subsystem66 ==
  BLU_FnBTPhoneDvcUp : TriggerPort  TriggerType=function-call  IsSimulinkFunction=on  FunctionName=BLU_FnBTPhoneDvcUp  VariantControl=(inherit)

== system ButtonLogic/ButtonStates/fnCallSubsystem/Function-Call Subsystem67 ==
  BLU_FnBTPhoneDvcDwn : TriggerPort  TriggerType=function-call  IsSimulinkFunction=on  FunctionName=BLU_FnBTPhoneDvcDwn  VariantControl=(inherit)

== system ButtonLogic/ButtonStates/fnCallSubsystem/Function-Call Subsystem68 ==
  BLU_FnBTHeadsetDvcUp : TriggerPort  TriggerType=function-call  IsSimulinkFunction=on  FunctionName=BLU_FnBTHeadsetDvcUp  VariantControl=(inherit)

== system ButtonLogic/ButtonStates/fnCallSubsystem/Function-Call Subsystem69 ==
  BLU_FnBTHeadsetDvcDwn : TriggerPort  TriggerType=function-call  IsSimulinkFunction=on  FunctionName=BLU_FnBTHeadsetDvcDwn  VariantControl=(inherit)

== system ButtonLogic/ButtonStates/fnCallSubsystem/Function-Call Subsystem7 ==
  BLU_FnBIWarningsDwn : TriggerPort  TriggerType=function-call  IsSimulinkFunction=on  FunctionName=BLU_FnBIWarningsDwn  VariantControl=(inherit)

== system ButtonLogic/ButtonStates/fnCallSubsystem/Function-Call Subsystem70 ==
  BLU_FnBTPhoneDvcDel : TriggerPort  TriggerType=function-call  IsSimulinkFunction=on  FunctionName=BLU_FnBTPhoneDvcDel  VariantControl=(inherit)

== system ButtonLogic/ButtonStates/fnCallSubsystem/Function-Call Subsystem71 ==
  BLU_FnBTHeadsetDvcDel : TriggerPort  TriggerType=function-call  IsSimulinkFunction=on  FunctionName=BLU_FnBTHeadsetDvcDel  VariantControl=(inherit)

== system ButtonLogic/ButtonStates/fnCallSubsystem/Function-Call Subsystem72 ==
  BLU_FnBTPhonePassKeyChkd : TriggerPort  TriggerType=function-call  IsSimulinkFunction=on  FunctionName=BLU_FnBTPhonePassKeyChkd  VariantControl=(inherit)

== system ButtonLogic/ButtonStates/fnCallSubsystem/Function-Call Subsystem73 ==
  BLU_FnBTPhonePairReq : TriggerPort  TriggerType=function-call  IsSimulinkFunction=on  FunctionName=BLU_FnBTPhonePairReq  VariantControl=(inherit)

== system ButtonLogic/ButtonStates/fnCallSubsystem/Function-Call Subsystem74 ==
  BLU_FnBTHeadsetPairReq : TriggerPort  TriggerType=function-call  IsSimulinkFunction=on  FunctionName=BLU_FnBTHeadsetPairReq  VariantControl=(inherit)

== system ButtonLogic/ButtonStates/fnCallSubsystem/Function-Call Subsystem75 ==
  BLU_FnCnctvtyCnfrmAppReg : TriggerPort  TriggerType=function-call  IsSimulinkFunction=on  FunctionName=BLU_FnCnctvtyCnfrmAppReg  VariantControl=(inherit)
  Terminator : Terminator
  u : ArgIn  ArgumentName=u
  wires:
  u/1 -> Terminator/1

== system ButtonLogic/ButtonStates/fnCallSubsystem/Function-Call Subsystem76 ==
  BLU_FnHdstSelCord : TriggerPort  TriggerType=function-call  IsSimulinkFunction=on  FunctionName=BLU_FnHdstSelCord  VariantControl=(inherit)

== system ButtonLogic/ButtonStates/fnCallSubsystem/Function-Call Subsystem77 ==
  BLU_FnHdstSelBT : TriggerPort  TriggerType=function-call  IsSimulinkFunction=on  FunctionName=BLU_FnHdstSelBT  VariantControl=(inherit)

== system ButtonLogic/ButtonStates/fnCallSubsystem/Function-Call Subsystem78 ==
  BLU_FnActvCallEXIT : TriggerPort  TriggerType=function-call  IsSimulinkFunction=on  FunctionName=BLU_FnActvCallEXIT  VariantControl=(inherit)

== system ButtonLogic/ButtonStates/fnCallSubsystem/Function-Call Subsystem79 ==
  BLU_FnLapTmrScrllUP : TriggerPort  TriggerType=function-call  IsSimulinkFunction=on  FunctionName=BLU_FnLapTmrScrllUP  VariantControl=(inherit)

== system ButtonLogic/ButtonStates/fnCallSubsystem/Function-Call Subsystem8 ==
  BLU_FnCCSwtONSpdLmtr : TriggerPort  TriggerType=function-call  IsSimulinkFunction=on  FunctionName=BLU_FnCCSwtONSpdLmtr  VariantControl=(inherit)

== system ButtonLogic/ButtonStates/fnCallSubsystem/Function-Call Subsystem80 ==
  BLU_FnActvCallSET : TriggerPort  TriggerType=function-call  IsSimulinkFunction=on  FunctionName=BLU_FnActvCallSET  VariantControl=(inherit)

== system ButtonLogic/ButtonStates/fnCallSubsystem/Function-Call Subsystem81 ==
  BLU_FnLapTmrScrllDOWN : TriggerPort  TriggerType=function-call  IsSimulinkFunction=on  FunctionName=BLU_FnLapTmrScrllDOWN  VariantControl=(inherit)

== system ButtonLogic/ButtonStates/fnCallSubsystem/Function-Call Subsystem9 ==
  BLU_FnCCSwtOFFSpdLmtr : TriggerPort  TriggerType=function-call  IsSimulinkFunction=on  FunctionName=BLU_FnCCSwtOFFSpdLmtr  VariantControl=(inherit)

== stateflow chart ButtonLogic/ButtonStates/fnCallSubsystem/Function-Call Subsystem36/Chart ==
  (default) -> (junction 1)
  (junction 1) -> (junction 3) [order 1] : [u == eStateName.CONSUMPTION_LTR_PER_100KM]
  (junction 3) -> (junction 5) : {y=0;}
  (junction 1) -> (junction 7) [order 2]
  (junction 5) -> (junction 11)
  (junction 7) -> (junction 9) [order 1] : [u == eStateName.CONSUMPTION_KM_PER_LTR]
  (junction 9) -> (junction 11) : {y=1;}
  (junction 7) -> (junction 14) [order 2]
  (junction 11) -> (junction 18)
  (junction 14) -> (junction 16) [order 1] : [u == eStateName.CONSUMPTION_USG_PER_100MI]
  (junction 16) -> (junction 18) : {y=2;}
  (junction 14) -> (junction 21) [order 2]
  (junction 18) -> (junction 25)
  (junction 23) -> (junction 25) : {y=3; }
  (junction 21) -> (junction 23) [order 1] : [u == CONSUMPTION_MI_PER_USG]
  (junction 25) -> (junction 32)
  (junction 21) -> (junction 28) [order 2]
  (junction 28) -> (junction 30) [order 1] : [u==CONSUMPTION_MI_PER_LTR]
  (junction 30) -> (junction 32) : {y=4;}
  (junction 28) -> (junction 35) [order 2]
  (junction 32) -> (junction 39)
  (junction 37) -> (junction 39) : {y=5;}
  (junction 35) -> (junction 37) [order 1] : [u == CONSUMPTION_UKG_PER_100MI]
  (junction 39) -> (junction 46)
  (junction 35) -> (junction 42) [order 2]
  (junction 44) -> (junction 46) : {y=6;}
  (junction 42) -> (junction 44) [order 1] : [u==CONSUMPTION_MI_PER_UKG]
  (junction 46) -> (junction 52)
  (junction 42) -> (junction 50) [order 2]
  (junction 52) -> (junction 50)
  data: y output uint16; u input
